simulink model "rolling_mill"  (Simulink 4.00)
settings: Solver=ode45  StartTime=0.0  StopTime=500  RelTol=1e-3
PreLoadFcn:
  | load rolling_mill
values from neighbouring files (symbols this model uses):
  gx = 1e-6    (= 1e-06)    [milldemo_sls.m]
  gxy = 0.1    [milldemo_sls.m]
  gy = 0.5e-6    (= 5e-07)    [milldemo_sls.m]
  gyx = 0.4    [milldemo_sls.m]
libraries: cstblocks x9, simulink3 x6
settings Model: Creator=pascal  LastModifiedBy=pascal  BlockReductionOpt=off

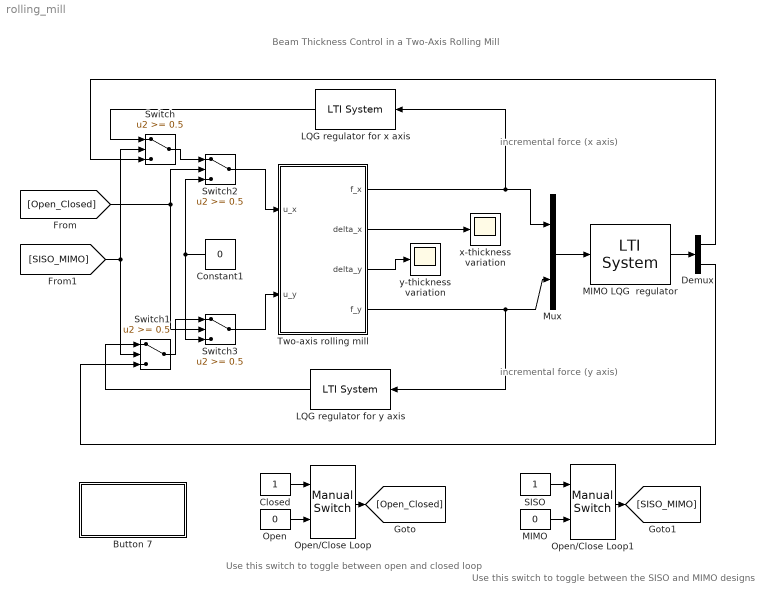
== system rolling_mill ==
  note: incremental force
      | (x axis)
  note: Use this switch to toggle between
      | open and closed loop
  note: Use this switch to toggle between
      | the SISO and MIMO designs
  note: Beam Thickness Control in a Two-Axis Rolling Mill
  note: incremental force
      | (y axis)
  Button 7 : Subsystem
      settings: OpenFcn=milldemo_sls  RTWFcnNameOpts=Auto  RTWFileNameOpts=Auto
      mask Display: disp('Double click here\nfor details\nabout the design')
  Closed : Constant  Value=1
  Constant1 : Constant  Orientation=left  Value=0
  Demux : Demux  Outputs=2  BusSelectionMode=off
  LQG regulator for x axis : cstblocks/LTI System  Orientation=left  sys=Regx  IC=0
  LQG regulator for y axis : cstblocks/LTI System  Orientation=left  sys=Regy  IC=0
  MIMO : Constant  Value=0
  "MIMO LQG  regulator " : cstblocks/LTI System  sys=Regxy  IC=0
  Mux : Mux  Inputs=2
  Open : Constant  Value=0
  Open/Close Loop : simulink3/Nonlinear/Manual Switch  sw=0  action=0
  Open/Close Loop1 : simulink3/Nonlinear/Manual Switch  sw=1  action=0
  SISO : Constant  Value=1
  Switch{,1..3} (4 alike) : Switch  Threshold=0.5
  Two-axis rolling mill : Subsystem
      settings: RTWFcnNameOpts=Auto  RTWFileNameOpts=Auto
  x-thickness variation : Scope
      settings: TimeRange=20  YMin=-0.8  YMax=0.8  SaveToWorkspace=off  SaveName=ScopeData  LimitDataPoints=on  MaxDataPoints=10000
  y-thickness variation : Scope
      settings: TimeRange=20  YMin=-0.8  YMax=0.6  SaveToWorkspace=off  LimitDataPoints=on  MaxDataPoints=10000
  wires:
  Two-axis rolling mill/4(f_y) -> LQG regulator for y axis/1, Mux/2
  Two-axis rolling mill/3(delta_y) -> y-thickness variation/1
  Two-axis rolling mill/1(f_x) -> LQG regulator for x axis/1, Mux/1
  LQG regulator for x axis/1 -> Switch/1
  LQG regulator for y axis/1 -> Switch1/1
  Mux/1 -> "MIMO LQG  regulator "/1
  Switch/1 -> Switch2/1
  Switch2/1 -> Two-axis rolling mill/1(u_x)
  "MIMO LQG  regulator "/1 -> Demux/1
  Demux/1 -> Switch/3
  Demux/2 -> Switch1/3
  Switch3/1 -> Two-axis rolling mill/2(u_y)
  Switch1/1 -> Switch3/1
  Closed/1 -> Open/Close Loop/1
  Constant1/1 -> Switch2/3, Switch3/3
  Open/1 -> Open/Close Loop/2
  Open/Close Loop/1 -> [Open_Closed]
  SISO/1 -> Open/Close Loop1/1
  MIMO/1 -> Open/Close Loop1/2
  Open/Close Loop1/1 -> [SISO_MIMO]
  [Open_Closed] -> Switch2/2, Switch3/2
  [SISO_MIMO] -> Switch/2, Switch1/2
  Two-axis rolling mill/2(delta_x) -> x-thickness variation/1

== system rolling_mill/Button 7 ==

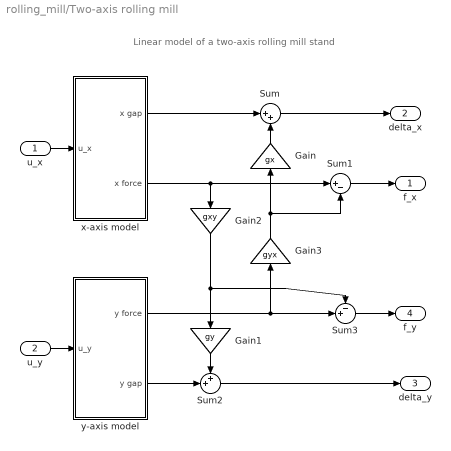
== system rolling_mill/Two-axis rolling mill ==
  note: Linear model of a two-axis rolling mill stand
  u_x : Inport  Port=1
  u_y : Inport  Port=2
  Gain : Gain  Orientation=up  Gain=gx  Multiplication=Element-wise(K.*u)  SaturateOnIntegerOverflow=on
  Gain1 : Gain  Orientation=down  Gain=gy  Multiplication=Element-wise(K.*u)  SaturateOnIntegerOverflow=on
  Gain2 : Gain  Orientation=down  Gain=gxy  Multiplication=Element-wise(K.*u)  SaturateOnIntegerOverflow=on
  Gain3 : Gain  Orientation=up  Gain=gyx  Multiplication=Element-wise(K.*u)  SaturateOnIntegerOverflow=on
  Sum : Sum  Inputs=|++  SaturateOnIntegerOverflow=on
  Sum1 : Sum  Inputs=|+-  SaturateOnIntegerOverflow=on
  Sum2 : Sum  Inputs=++|  SaturateOnIntegerOverflow=on
  Sum3 : Sum  Inputs=-+|  SaturateOnIntegerOverflow=on
  x-axis model : Subsystem
      settings: RTWFcnNameOpts=Auto  RTWFileNameOpts=Auto
  y-axis model : Subsystem
      settings: RTWFcnNameOpts=Auto  RTWFileNameOpts=Auto
  f_x : Outport  Port=1
  delta_x : Outport  Port=2
  delta_y : Outport  Port=3
  f_y : Outport  Port=4
  wires:
  x-axis model/1(x gap) -> Sum/1
  Gain/1 -> Sum/2
  x-axis model/2(x force) -> Sum1/1, Gain2/1
  y-axis model/2(y gap) -> Sum2/2
  Gain1/1 -> Sum2/1
  Gain2/1 -> Gain1/1, Sum3/1
  y-axis model/1(y force) -> Sum3/2, Gain3/1
  Sum/1 -> delta_x/1
  u_x/1 -> x-axis model/1(u_x)
  Sum1/1 -> f_x/1
  Sum3/1 -> f_y/1
  u_y/1 -> y-axis model/1(u_y)
  Sum2/1 -> delta_y/1
  Gain3/1 -> Gain/1, Sum1/2

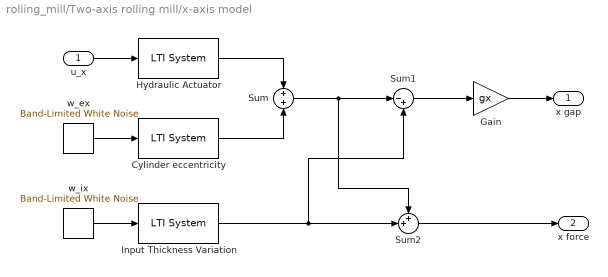
== system rolling_mill/Two-axis rolling mill/x-axis model ==
  u_x : Inport  Port=1
  Cylinder eccentricity : cstblocks/LTI System  sys=Fex  IC=0
  Gain : Gain  Gain=gx  Multiplication=Element-wise(K.*u)  SaturateOnIntegerOverflow=on
  Hydraulic Actuator : cstblocks/LTI System  sys=Hx  IC=0
  Input Thickness Variation : cstblocks/LTI System  sys=Fix  IC=0
  Sum : Sum  Inputs=++  SaturateOnIntegerOverflow=on
  Sum1 : Sum  Inputs=|-+  SaturateOnIntegerOverflow=on
  Sum2 : Sum  Inputs=++|  SaturateOnIntegerOverflow=on
  w_ex : simulink3/Sources/Band-Limited White Noise  Cov=sqrt(1/0.01)  Ts=0.01  seed=[23341]
  w_ix : simulink3/Sources/Band-Limited White Noise  Cov=sqrt(1/0.01)  Ts=0.01  seed=[23341]
  x gap : Outport  Port=1
  x force : Outport  Port=2
  wires:
  w_ex/1 -> Cylinder eccentricity/1
  u_x/1 -> Hydraulic Actuator/1
  Hydraulic Actuator/1 -> Sum/1
  Cylinder eccentricity/1 -> Sum/2
  Sum/1 -> Sum1/1, Sum2/1
  Sum1/1 -> Gain/1
  w_ix/1 -> Input Thickness Variation/1
  Input Thickness Variation/1 -> Sum2/2, Sum1/2
  Gain/1 -> x gap/1
  Sum2/1 -> x force/1

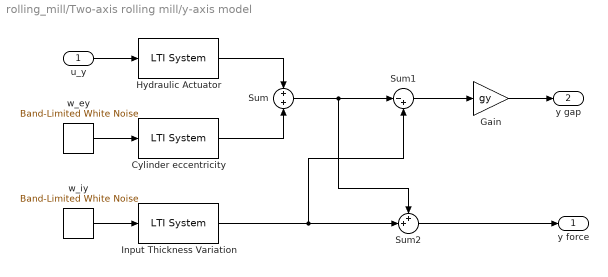
== system rolling_mill/Two-axis rolling mill/y-axis model ==
  u_y : Inport  Port=1
  Cylinder eccentricity : cstblocks/LTI System  sys=Fey  IC=0
  Gain : Gain  Gain=gy  Multiplication=Element-wise(K.*u)  SaturateOnIntegerOverflow=on
  Hydraulic Actuator : cstblocks/LTI System  sys=Hy  IC=0
  Input Thickness Variation : cstblocks/LTI System  sys=Fiy  IC=0
  Sum : Sum  Inputs=++  SaturateOnIntegerOverflow=on
  Sum1 : Sum  Inputs=|-+  SaturateOnIntegerOverflow=on
  Sum2 : Sum  Inputs=++|  SaturateOnIntegerOverflow=on
  w_ey : simulink3/Sources/Band-Limited White Noise  Cov=sqrt(1/0.01)  Ts=0.01  seed=[23341]
  w_iy : simulink3/Sources/Band-Limited White Noise  Cov=sqrt(1/0.01)  Ts=0.01  seed=[23341]
  y force : Outport  Port=1
  y gap : Outport  Port=2
  wires:
  Sum2/1 -> y force/1
  Gain/1 -> y gap/1
  Input Thickness Variation/1 -> Sum1/2, Sum2/2
  w_iy/1 -> Input Thickness Variation/1
  Sum1/1 -> Gain/1
  Sum/1 -> Sum2/1, Sum1/1
  Cylinder eccentricity/1 -> Sum/2
  Hydraulic Actuator/1 -> Sum/1
  u_y/1 -> Hydraulic Actuator/1
  w_ey/1 -> Cylinder eccentricity/1
